simulink model "pdf_subsis2"  (R2023a)
settings: Solver=VariableStepAuto  StartTime=0.0  StopTime=10.0  RelTol=1e-3
values from neighbouring files (symbols this model uses):
  TABLEDATA = [1.10335162023 0.00823171458117 -11.0555848055 -0.375153780134 6.18853169798 -34.1001082535 0.0324757076966 -9.89122049893 0.729242255451 -0.683674300952 1.08721495624 0.00509823507416 ... (12710 elements, 2x5x41x31)]    [TableData_002.mat]    (also in TableData_004.mat = [0.174322085341 -0.0514346863342 -0.753716023023 2.529946466; TableData_006.mat = [0.237084016899 -0.0298197541441 -1.42090322153 1.5613882815; TableData_007GS.mat = [0.237084016899 -0.0298197541441 -1.42090322153 1.5613882815; TableData_009.mat = [0.235717817503 -0.0298554739715 -1.40805314109 1.5648466906)
libraries: simulink_extras x1
settings Model: Creator=ignac  LastModifiedBy=ignac

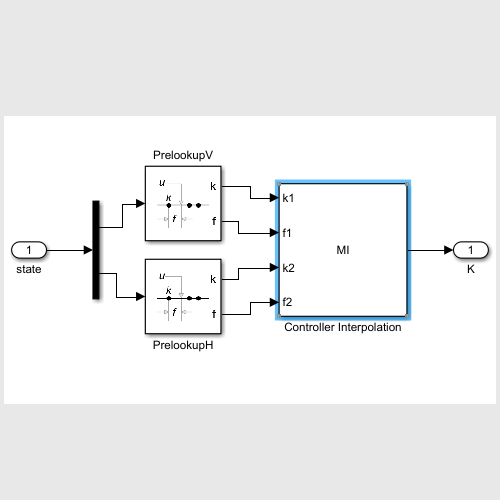
[thumbnail: Simulink's stored preview of the top-level diagram]
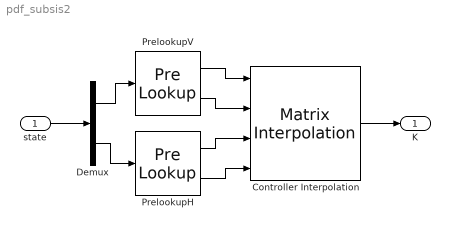
== system pdf_subsis2 ==
  state : Inport
  Controller Interpolation : simulink_extras/Additional Lookup Tables/Matrix Interpolation  InterpMethod=Linear  ExtrapMethod=Clip  InterpolateDimension=2  TableData=TABLEDATA  SimulateUsing=Code generation
  Demux : Demux  Outputs=2
  PrelookupH : PreLookup  BreakpointsData=vH  ExtrapMethod=Linear
  PrelookupV : PreLookup  BreakpointsData=vV  ExtrapMethod=Linear
  K : Outport
  wires:
  PrelookupV/2 -> Controller Interpolation/2
  Demux/1 -> PrelookupV/1
  Demux/2 -> PrelookupH/1
  state/1 -> Demux/1
  Controller Interpolation/1 -> K/1
  PrelookupH/1 -> Controller Interpolation/3
  PrelookupV/1 -> Controller Interpolation/1
  PrelookupH/2 -> Controller Interpolation/4
